simulink model "UAV_sync_known_sim_wrong_version"  (R2018b)
settings: Solver=ode23tb  StartTime=0.0  StopTime=35
values from neighbouring files (symbols this model uses):
  C_rho = 1.225    [SC42120_UAV_Preconditions.m]
  D0 = [M0 0 0 0 0 0 ... (first row only)    [SC42120_UAV_Preconditions.m]
  D1 = [eye(3)*M1 zeros(3,3) ... (first row only)    [UAV_sync_known.m]    (also in UAV_sync_unknown.m; UAV_sync_unknown_gap.m)
  D2 = [eye(3)*M2 zeros(3,3) ... (first row only)    [UAV_sync_known.m]    (also in UAV_sync_unknown.m; UAV_sync_unknown_gap.m)
  Derivative_gain_phi = 50    [SC42120_UAV_Preconditions.m]
  Derivative_gain_psi = 50    [SC42120_UAV_Preconditions.m]
  Derivative_gain_theta = 50    [SC42120_UAV_Preconditions.m]
  Derivative_gain_x = 50    [SC42120_UAV_Preconditions.m]
  Derivative_gain_y = 50    [SC42120_UAV_Preconditions.m]
  Derivative_gain_z = 50    [SC42120_UAV_Preconditions.m]
  G = 9.80665    [SC42120_UAV_Preconditions.m]
  g0 = [0;0;-M0*G;0;0;0]    [SC42120_UAV_Preconditions.m]
  I0 = [0.02 0 -0.01 ... (first row only)    [SC42120_UAV_Preconditions.m]
  I1 = [0.1 0 -0.01 ... (first row only)    [UAV_sync_known.m]    (also in UAV_sync_unknown.m; UAV_sync_unknown_gap.m)
  I2 = 2*[0.1 0 -0.01 ... (first row only)    [UAV_sync_known.m]    (also in UAV_sync_unknown.m; UAV_sync_unknown_gap.m)
  InitWind = [0;0;0]    [SC42120_UAV_Preconditions.m]
  Kp = diag(P)    [SC42120_UAV_Preconditions.m]
  Kv = diag(V)    [SC42120_UAV_Preconditions.m]
  M0 = 10    [SC42120_UAV_Preconditions.m]
  M1 = 20    [UAV_sync_known.m]    (also in UAV_sync_unknown.m; UAV_sync_unknown_gap.m)
  M2 = 30    [UAV_sync_known.m]    (also in UAV_sync_unknown.m; UAV_sync_unknown_gap.m)
  Proportional_phi = 50    [SC42120_UAV_Preconditions.m]
  Proportional_psi = 50    [SC42120_UAV_Preconditions.m]
  Proportional_theta = 50    [SC42120_UAV_Preconditions.m]
  Proportional_x = 50    [SC42120_UAV_Preconditions.m]
  Proportional_y = 50    [SC42120_UAV_Preconditions.m]
  Proportional_z = 50    [SC42120_UAV_Preconditions.m]
undefined symbols (not defined in the file or in its folder): Aero, APlane, Bxl, C, Ctr, deg, DiscIntNeverNeededParam, F, Guid, Init, Light, MIL, Path, rad, s, Trim, Utility
libraries: aerolibconvert2 x37, simulink x15, dspsigops x7, shared6dof x4, aerolibasang x4, sharedutil x4, simulink_extras x3, aerolibadyn x1, aerolibtransform2 x1, aerolibwind2 x1
(part 4 of 6)

== system UAV_sync_known_sim_wrong_version/Node 0/VF Approach/AUTOPILOT/Low-level Controllers/Pitch controller/TRASH ==
  Abs : Abs  Commented=on
  Angle Conversion2 : aerolibconvert2/Angle Conversion  Commented=on  IU=rad  OU=deg
  Angle Conversion3 : aerolibconvert2/Angle Conversion  Commented=on  IU=rad  OU=deg
  Coordination_offset_MATLAB_Fcn : MATLAB Function  Commented=on  TreatAsAtomicUnit=on
  Digital Clock : DigitalClock  Commented=on  SampleTime=0.001
  From : From  Commented=on  GotoTag=roll_ang
  From1 : From  Commented=on  GotoTag=Va  TagVisibility=global
  From2 : From  Commented=on  GotoTag=Va  TagVisibility=global
  From3 : From  Commented=on  GotoTag=pitch_ang
  From5 : From  Commented=on  GotoTag=pitch_ang
  From6 : From  Commented=on  GotoTag=Va  TagVisibility=global
  From7 : From  Commented=on  GotoTag=pitch_ang
  If : If  Commented=on  IfExpression=u1 > 70
  If Action Subsystem : Subsystem  Commented=on  TreatAsAtomicUnit=on
  If Action Subsystem1 : Subsystem  Commented=on  TreatAsAtomicUnit=on
  Merge : Merge  Commented=on
  Parameters mixer1 : Subsystem  Commented=on
  Parameters mixer2 : Subsystem  Commented=on
  Pitch_PID_MATLAB_Fcn : MATLAB Function  Commented=on  TreatAsAtomicUnit=on
  Saturation : Saturate  Commented=on  UpperLimit=80  LowerLimit=-80
  Terminator : Terminator  Commented=on
  wires:
  Parameters mixer2/1(parameters_roll_comp) -> Coordination_offset_MATLAB_Fcn/4(parameters)
  From2/1 -> Coordination_offset_MATLAB_Fcn/3(aspeed)
  From3/1 -> Coordination_offset_MATLAB_Fcn/2(meas_pitch_angle)
  Angle Conversion2/1 -> Coordination_offset_MATLAB_Fcn/1(bank_angle)
  From7/1 -> Abs/1
  Saturation/1 -> If Action Subsystem1/2(bank)
  From5/1 -> If Action Subsystem1/1(pitch)
  From/1 -> Angle Conversion3/1
  If Action Subsystem/1(Out1) -> Merge/1
  If/2 -> If Action Subsystem1/Action
  Angle Conversion3/1 -> Saturation/1
  If/1 -> If Action Subsystem/Action
  Merge/1 -> Terminator/1  "rate offset"
  From6/1 -> If Action Subsystem1/3(Va)
  If Action Subsystem1/1(Out1) -> Merge/2
  Abs/1 -> If/1

== system UAV_sync_known_sim_wrong_version/Node 0/VF Approach/AUTOPILOT/Low-level Controllers/Roll controller/Roll Rate Controller ==
  Desidered rate : Inport
  Roll Rate : Inport  Port=2
  Scaler : Inport  Port=3
  +-45 : Saturate  UpperLimit=45  LowerLimit=-45
  Anti-windup : Subsystem
  Constant4 : Constant  Value=Ctr.Roll.RLL2SRV_I
  Constant8 : Constant  Value=Ctr.Roll.RLL2SRV_D
  Constant9 : Constant  Value=Ctr.TS
  IMAX(deg) : Saturate  UpperLimit=Ctr.Roll.RLL2SRV_IMAX_SCALED  LowerLimit=-Ctr.Roll.RLL2SRV_IMAX_SCALED
  K_FF (real feedforward) : Subsystem
  K_P (feedforward) : Subsystem
  Product2 : Product  Inputs=**
  Product3 : Product  Inputs=****
  Product4 : Product  Inputs=***
  Product5 : Product  Inputs=***
  Product6 : Product  Inputs=***
  Scaler_1 : InportShadow  Port=3
  Scaler_2 : InportShadow  Port=3
  Scaler_3 : InportShadow  Port=3
  Sum2 : Sum  Inputs=|+-
  Sum3 : Sum  Inputs=++++
  Sum5 : Sum  Inputs=++|
  Tau1 : Gain  Gain=Ctr.Roll.RLL2SRV_TCONST
  Unit Delay1 : UnitDelay  SampleTime=Ctr.TS
  Unit Delay2 : UnitDelay  SampleTime=Ctr.TS
  Ail_dem : Outport
  wires:
  Anti-windup/1(y_int) -> Sum5/2
  Product3/1 -> Anti-windup/2(u)  "integrator_delta"
  Unit Delay1/1 -> Sum5/1
  Constant8/1 -> Product5/2
  Product4/1 -> Sum3/2  "PID_P"
  Scaler_3/1 -> Product4/3
  Scaler_2/1 -> Product6/3
  [DesRate] -> Product6/2
  Product2/1 -> [rateErr], Product3/1  "rate_error"
  Roll Rate/1 -> Sum2/2
  Sum2/1 -> Product2/1
  Constant9/1 -> Product3/3
  Scaler/1 -> Product2/2, Product3/4
  IMAX(deg)/1 -> Sum3/1, Unit Delay1/1  "PID_I"
  [rateErr] -> Product5/1
  Product5/1 -> Sum3/3  "PID_D"
  Constant4/1 -> Tau1/1
  Tau1/1 -> Product3/2  "ki_rate"
  Sum3/1 -> Unit Delay2/1, +-45/1
  [DesRate] -> Product4/2
  Scaler_1/1 -> Product5/3
  Product6/1 -> Sum3/4  "PID_FF"
  Unit Delay2/1 -> Anti-windup/1(y)
  Sum5/1 -> IMAX(deg)/1
  +-45/1 -> Ail_dem/1
  Desidered rate/1 -> [DesRate], Sum2/1
  K_P (feedforward)/1(Out1) -> Product4/1
  K_FF (real feedforward)/1(Out1) -> Product6/1

== system UAV_sync_known_sim_wrong_version/Node 0/VF Approach/AUTOPILOT/Low-level Controllers/Roll controller/Roll Rate Controller (simpl. continuous) ==
  Roll Rate Error : Inport
  Roll rate : Inport  Port=2
  Scaler : Inport  Port=3
  Ctr.Roll.RLL2SRV_D : Gain  Gain=Ctr.Roll.RLL2SRV_D
  Integrator : Integrator
  Kp : Gain  Gain=Ctr.Roll.K_P
  Product : Product
  Product1 : Product
  Sum1 : Sum  Inputs=|+-
  Sum2 : Sum  Inputs=+++
  k_I : Gain  Gain=Ctr.Roll.K_I
  AilDemand : Outport
  wires:
  Roll Rate Error/1 -> Sum1/1, Kp/1
  Roll rate/1 -> Sum1/2
  Integrator/1 -> Sum2/3
  Product1/1 -> AilDemand/1
  Product/1 -> k_I/1, Ctr.Roll.RLL2SRV_D/1
  Ctr.Roll.RLL2SRV_D/1 -> Sum2/2
  Sum1/1 -> Product/1
  Scaler/1 -> Product/2, Product1/2
  Kp/1 -> Sum2/1
  k_I/1 -> Integrator/1
  Sum2/1 -> Product1/1

== system UAV_sync_known_sim_wrong_version/Node 0/VF Approach/AUTOPILOT/Low-level Controllers/Side-slip angle controller/Coordination offset ==
  note: Coordinated Turn
  Bank : Inport
  Constant1 : Constant  Value=Ctr.Yaw.YAW2SRV_RLL
  Constant6 : Constant  Value=APlane.airspeed_min
  Constant8 : Constant  Value=C.g
  MinMax : MinMax  Function=max  Inputs=2
  Product1 : Product  Inputs=*/
  Product2 : Product  Inputs=****
  Trigonometric Function : Trigonometry  Operator=tan
  Trigonometric Function1 : Trigonometry  Operator=cos
  yaw_rate_correction : Outport
  wires:
  Constant8/1 -> Product1/1
  [Va] -> MinMax/1
  Constant6/1 -> MinMax/2
  MinMax/1 -> Product1/2
  Product1/1 -> Product2/1
  Trigonometric Function/1 -> Product2/2
  Constant1/1 -> Product2/4
  Bank/1 -> Trigonometric Function1/1, Trigonometric Function/1  "roll angle"
  Trigonometric Function1/1 -> Product2/3
  Product2/1 -> yaw_rate_correction/1

== system UAV_sync_known_sim_wrong_version/Node 0/VF Approach/AUTOPILOT/Low-level Controllers/Side-slip angle controller/High-Pass Filter ==
  note: Highpass filter with cutoff frequency at 0.2 rad/s
  In : Inport
  Gain : Gain  Gain=0.9960080
  Scope : Scope  NumInputPorts=2
  Sum3 : Sum  Inputs=++|
  Sum4 : Sum  Inputs=-+|
  Unit Delay : UnitDelay  SampleTime=Ctr.TS
  Unit Delay1 : UnitDelay  SampleTime=Ctr.TS
  Out : Outport
  wires:
  Unit Delay/1 -> Gain/1
  Sum4/1 -> Sum3/1
  Sum3/1 -> Unit Delay/1, Scope/2, Out/1
  Unit Delay1/1 -> Sum4/1
  Gain/1 -> Sum3/2
  In/1 -> Scope/1, Unit Delay1/1, Sum4/2

== system UAV_sync_known_sim_wrong_version/Node 0/VF Approach/BIXLER DYNAMICS/RUBBISH BIN/Orbit/Chi_d ==
  gamma : Inport
  j : Inport  Port=2
  d : Inport  Port=3
  r : Inport  Port=4
  k : Inport  Port=5
  Vector Field (loiter) : MATLAB Function  TreatAsAtomicUnit=on
  chi_d : Outport
  d_tilde : Outport  Port=2
  wires:
  gamma/1 -> Vector Field (loiter)/1(gamma)
  Vector Field (loiter)/2(d_tilde) -> d_tilde/1
  Vector Field (loiter)/1(chi_d) -> chi_d/1
  k/1 -> Vector Field (loiter)/5(k)
  d/1 -> Vector Field (loiter)/3(d)
  r/1 -> Vector Field (loiter)/4(radius)
  j/1 -> Vector Field (loiter)/2(j)

== system UAV_sync_known_sim_wrong_version/Node 0/VF Approach/BIXLER DYNAMICS/RUBBISH BIN/Orbit/Compute gamma ==
  xy : Inport
  OrbitCenter : Inport  Port=2
  chi : Inport  Port=3
  Demux : Demux  Outputs=2
  L.PolarCoord : MATLAB Function  TreatAsAtomicUnit=on
  Unwrap : dspsigops/Unwrap  tol=pi  running=off
  Zero-Order Hold{2..5} (4 alike) : ZeroOrderHold  SampleTime=-1
  gamma : Outport
  d : Outport  Port=2
  wires:
  Demux/2 -> Zero-Order Hold3/1
  OrbitCenter/1 -> Zero-Order Hold4/1
  L.PolarCoord/2(d) -> d/1
  L.PolarCoord/1(gamma) -> Unwrap/1
  xy/1 -> Demux/1
  Zero-Order Hold2/1 -> L.PolarCoord/1(x)
  Demux/1 -> Zero-Order Hold2/1
  chi/1 -> Zero-Order Hold5/1
  Zero-Order Hold5/1 -> L.PolarCoord/4(chi)
  Zero-Order Hold3/1 -> L.PolarCoord/2(y)
  Zero-Order Hold4/1 -> L.PolarCoord/3(c)
  Unwrap/1 -> gamma/1

== system UAV_sync_known_sim_wrong_version/Node 0/VF Approach/BIXLER DYNAMICS/RUBBISH BIN/Orbit/Extract Vg(xy). ==
  In1 : Inport
  Demux : Demux  Outputs=2
  Math Function : Math  Operator=hypot  SaturateOnIntegerOverflow=on
  Selector3 : Selector  InputPortWidth=3  IndexOptions=Index vector (dialog)  Indices=[1 2]  OutputSizes=1
  Out1 : Outport
  wires:
  In1/1 -> Selector3/1
  Math Function/1 -> Out1/1  "V_g"
  Demux/2 -> Math Function/2
  Selector3/1 -> Demux/1
  Demux/1 -> Math Function/1

== system UAV_sync_known_sim_wrong_version/Node 0/VF Approach/BIXLER DYNAMICS/RUBBISH BIN/Orbit/Loiter Controller ==
  chi : Inport
  chi_d : Inport  Port=2
  d : Inport  Port=3
  Vg_hat : Inport  Port=4
  gamma : Inport  Port=5
  Vg : Inport  Port=6
  param : Inport  Port=7
  Beard Version : MATLAB Function  TreatAsAtomicUnit=on
  Constant : Constant  Value=Guid.Method
  Loiter Controller : MATLAB Function  TreatAsAtomicUnit=on
  Manual Switch1 : ManualSwitch  CurrentSetting=0
  Scope : Scope
  Scope1 : Scope
  Scope10 : Scope  NumInputPorts=2
  Scope4 : Scope
  Switch : Switch  Criteria=u2 > Threshold  Threshold=0.5
  chi:_c : Outport
  wires:
  Loiter Controller/3(beta) -> Scope1/1
  Loiter Controller/5(term3) -> Scope10/2
  Loiter Controller/2(err) -> Scope/1
  Loiter Controller/4(term2) -> Scope10/1, Scope4/1
  chi_d/1 -> Loiter Controller/2(chi_d), [chi_d]
  d/1 -> Beard Version/3(d), Loiter Controller/3(d)
  Vg_hat/1 -> Loiter Controller/4(Vg)
  chi/1 -> Beard Version/1(chi), Loiter Controller/1(chi)
  param/1 -> Beard Version/6(param), Loiter Controller/6(param)
  gamma/1 -> Beard Version/5(gamma), Loiter Controller/5(gamma)
  Constant/1 -> Switch/2
  Loiter Controller/1(y) -> Switch/1
  Beard Version/1(chi_c) -> Switch/3
  Switch/1 -> Manual Switch1/2
  [chi_d] -> Manual Switch1/1
  [chi_d] -> Beard Version/2(chi_d)
  Vg/1 -> Beard Version/4(Vg)
  Manual Switch1/1 -> chi:_c/1

== system UAV_sync_known_sim_wrong_version/Node 0/VF Approach/BIXLER DYNAMICS/RUBBISH BIN/Orbit/Parameters Mixer ==
  Constant1 : Constant  Value=Guid.Est.alpha
  Constant6 : Constant  Value=Guid.Loiter.k
  Constant7 : Constant  Value=Guid.Loiter.kk
  Constant8 : Constant  Value=Guid.Loiter.eps
  Mux : Mux  Inputs=6
  param : Outport
  wires:
  Mux/1 -> param/1
  Constant6/1 -> Mux/1
  Constant7/1 -> Mux/2
  Constant8/1 -> Mux/3
  [R] -> Mux/4
  [j] -> Mux/5
  Constant1/1 -> Mux/6

== system UAV_sync_known_sim_wrong_version/Node 0/VF Approach/BIXLER DYNAMICS/RUBBISH BIN/Orbit/Parameters Mixer1 ==
  Constant : Constant  Value=Guid.Wind.W
  Constant1 : Constant  Value=Guid.Loiter.phiw
  Constant11 : Constant  Value=Guid.Loiter.gamma
  Constant2 : Constant  Value=Guid.Loiter.d_int
  Constant3 : Constant  Value=Guid.Loiter.sigma
  Constant6 : Constant  Value=Guid.Loiter.k
  Constant7 : Constant  Value=Guid.Loiter.kk
  Constant8 : Constant  Value=Guid.Loiter.eps
  Mux : Mux  Inputs=11
  param : Outport
  wires:
  Constant11/1 -> Mux/10
  [R] -> Mux/8
  Mux/1 -> param/1
  [j] -> Mux/9
  Constant/1 -> Mux/1
  Constant8/1 -> Mux/6
  Constant6/1 -> Mux/4
  Constant7/1 -> Mux/5
  [Target_Airspeed] -> Mux/3
  Constant1/1 -> Mux/2
  Constant2/1 -> Mux/7
  Constant3/1 -> Mux/11

== system UAV_sync_known_sim_wrong_version/Node 0/VF Approach/BIXLER DYNAMICS/RUBBISH BIN/Orbit/Vg Estimator ==
  chi : Inport
  d : Inport  Port=2
  gamma : Inport  Port=3
  chi_d : Inport  Port=4
  param : Inport  Port=5
  vg : Inport  Port=6
  Reset : Inport  Port=7
  "Estimator " : MATLAB Function  TreatAsAtomicUnit=on
  Integrator1 : Integrator  ExternalReset=rising  InitialCondition=Guid.Vg0
  Scope16 : Scope  NumInputPorts=4
  Scope17 : Scope  NumInputPorts=3
  Vg_hat : Outport
  wires:
  "Estimator "/1(Vg2_hat_dot) -> Integrator1/1
  "Estimator "/8(chi_tilde) -> Scope17/3
  chi_d/1 -> "Estimator "/5(chi_d)
  "Estimator "/5(term2) -> Scope16/4
  "Estimator "/4(term1) -> Scope16/3
  Integrator1/1 -> Vg_hat/1, [Vg_hat]  "Vg_hat"
  [Vg_hat] -> "Estimator "/3(Vg_hat)
  "Estimator "/7(err_2) -> Scope17/2
  d/1 -> "Estimator "/2(d)
  "Estimator "/6(err_1) -> Scope17/1
  chi/1 -> "Estimator "/1(chi)
  "Estimator "/3(der) -> Scope16/2
  param/1 -> "Estimator "/6(param)
  "Estimator "/2(beta) -> Scope16/1
  gamma/1 -> "Estimator "/4(gamma)
  vg/1 -> "Estimator "/7(Vg)
  Reset/1 -> Integrator1/2

== system UAV_sync_known_sim_wrong_version/Node 0/VF Approach/BIXLER DYNAMICS/RUBBISH BIN/Reference Signals/Pitch Reference Generator ==
  Throttle : Inport
  Angle Conversion1 : aerolibconvert2/Angle Conversion  IU=deg  OU=rad
  "Ctr.Pitch.Trimmed " : Gain  Commented=on  Gain=Ctr.Pitch.Trimmed
  Step1 : Step  Time=Ctr.Gen.stepTimeElev  After=Ctr.Gen.stepElev  SampleTime=0
  Sum : Sum  Inputs=|++
  Pitch Reference : Outport
  wires:
  Step1/1 -> Sum/1
  Angle Conversion1/1 -> Pitch Reference/1  "Pitch Demand (rad)"
  "Ctr.Pitch.Trimmed "/1 -> Sum/2
  Sum/1 -> Angle Conversion1/1
  Throttle/1 -> "Ctr.Pitch.Trimmed "/1

== system UAV_sync_known_sim_wrong_version/Node 0/VF Approach/BIXLER DYNAMICS/RUBBISH BIN/Reference Signals/Roll Reference Generator ==
  Angle Conversion : aerolibconvert2/Angle Conversion  IU=deg  OU=rad
  Scope : Scope
  Step : Step  Commented=on  Time=Ctr.Gen.stepTimeAilFinal  After=-Ctr.Gen.stepAil  SampleTime=0
  Step1 : Step  Time=Ctr.Gen.stepTimeAil  After=Ctr.Gen.stepAil  SampleTime=0
  Step2 : Step  Commented=on  Time=Ctr.Gen.stepTimeAil+Ctr.Gen.stepAilDelay  After=-Ctr.Gen.stepAil  SampleTime=0
  Step3 : Step  Commented=on  Time=Ctr.Gen.stepTimeAilFinal+Ctr.Gen.stepAilDelay  After=Ctr.Gen.stepAil  SampleTime=0
  Sum : Sum  Inputs=++++
  RollDemand : Outport
  wires:
  Step3/1 -> Sum/4
  Step1/1 -> Sum/1
  Step/1 -> Sum/2
  Angle Conversion/1 -> RollDemand/1
  Step2/1 -> Sum/3
  Sum/1 -> Angle Conversion/1, Scope/1

== system UAV_sync_known_sim_wrong_version/Node 0/VF Approach/BIXLER DYNAMICS/RUBBISH BIN/Reference Signals/Yaw Reference Generator ==
  Angle Conversion : aerolibconvert2/Angle Conversion  IU=deg  OU=rad
  Scope : Scope
  Step : Step  Time=Ctr.Gen.stepTimeAilFinal  After=-Ctr.Gen.stepAil  SampleTime=0
  Step1 : Step  Time=Ctr.Gen.stepTimeAil  After=Ctr.Gen.stepAil  SampleTime=0
  Step2 : Step  Time=Ctr.Gen.stepTimeAil+Ctr.Gen.stepAilDelay  After=-Ctr.Gen.stepAil  SampleTime=0
  Step3 : Step  Time=Ctr.Gen.stepTimeAilFinal+Ctr.Gen.stepAilDelay  After=Ctr.Gen.stepAil  SampleTime=0
  Sum : Sum  Inputs=++++
  YawDemand : Outport
  wires:
  Step3/1 -> Sum/4
  Step1/1 -> Sum/1
  Step/1 -> Sum/2
  Angle Conversion/1 -> YawDemand/1
  Step2/1 -> Sum/3
  Sum/1 -> Angle Conversion/1, Scope/1

== system UAV_sync_known_sim_wrong_version/Node 0/VF Approach/BIXLER DYNAMICS/RUBBISH BIN/Reference Signals1/Pitch Reference Generator ==
  Throttle : Inport
  Angle Conversion1 : aerolibconvert2/Angle Conversion  IU=deg  OU=rad
  "Ctr.Pitch.Trimmed " : Gain  Commented=on  Gain=Ctr.Pitch.Trimmed
  Step1 : Step  Time=Ctr.Gen.stepTimeElev  After=Ctr.Gen.stepElev  SampleTime=0
  Sum : Sum  Inputs=|++
  Pitch Reference : Outport
  wires:
  Throttle/1 -> "Ctr.Pitch.Trimmed "/1
  Sum/1 -> Angle Conversion1/1
  "Ctr.Pitch.Trimmed "/1 -> Sum/2
  Angle Conversion1/1 -> Pitch Reference/1  "Pitch Demand (rad)"
  Step1/1 -> Sum/1

== system UAV_sync_known_sim_wrong_version/Node 0/VF Approach/BIXLER DYNAMICS/RUBBISH BIN/Reference Signals1/Roll Reference Generator ==
  Angle Conversion : aerolibconvert2/Angle Conversion  IU=deg  OU=rad
  Scope : Scope
  Step : Step  Commented=on  Time=Ctr.Gen.stepTimeAilFinal  After=-Ctr.Gen.stepAil  SampleTime=0
  Step1 : Step  Time=Ctr.Gen.stepTimeAil  After=Ctr.Gen.stepAil  SampleTime=0
  Step2 : Step  Commented=on  Time=Ctr.Gen.stepTimeAil+Ctr.Gen.stepAilDelay  After=-Ctr.Gen.stepAil  SampleTime=0
  Step3 : Step  Commented=on  Time=Ctr.Gen.stepTimeAilFinal+Ctr.Gen.stepAilDelay  After=Ctr.Gen.stepAil  SampleTime=0
  Sum : Sum  Inputs=++++
  RollDemand : Outport
  wires:
  Sum/1 -> Scope/1, Angle Conversion/1
  Step2/1 -> Sum/3
  Angle Conversion/1 -> RollDemand/1
  Step/1 -> Sum/2
  Step1/1 -> Sum/1
  Step3/1 -> Sum/4

== system UAV_sync_known_sim_wrong_version/Node 0/VF Approach/BIXLER DYNAMICS/RUBBISH BIN/Reference Signals1/Yaw Reference Generator ==
  Angle Conversion : aerolibconvert2/Angle Conversion  IU=deg  OU=rad
  Scope : Scope
  Step : Step  Time=Ctr.Gen.stepTimeAilFinal  After=-Ctr.Gen.stepAil  SampleTime=0
  Step1 : Step  Time=Ctr.Gen.stepTimeAil  After=Ctr.Gen.stepAil  SampleTime=0
  Step2 : Step  Time=Ctr.Gen.stepTimeAil+Ctr.Gen.stepAilDelay  After=-Ctr.Gen.stepAil  SampleTime=0
  Step3 : Step  Time=Ctr.Gen.stepTimeAilFinal+Ctr.Gen.stepAilDelay  After=Ctr.Gen.stepAil  SampleTime=0
  Sum : Sum  Inputs=++++
  YawDemand : Outport
  wires:
  Sum/1 -> Scope/1, Angle Conversion/1
  Step2/1 -> Sum/3
  Angle Conversion/1 -> YawDemand/1
  Step/1 -> Sum/2
  Step1/1 -> Sum/1
  Step3/1 -> Sum/4

== system UAV_sync_known_sim_wrong_version/Node 0/VF Approach/BIXLER DYNAMICS/RUBBISH BIN/Straight Line/Chi_d ==
  ey : Inport
  chi_q : Inport  Port=2
  chi_inf : Inport  Port=3
  k_line : Inport  Port=4
  Vector Field (straight line) : MATLAB Function  TreatAsAtomicUnit=on
  chi_d : Outport
  wires:
  chi_inf/1 -> Vector Field (straight line)/3(chi_inf)
  k_line/1 -> Vector Field (straight line)/4(k_line)
  ey/1 -> Vector Field (straight line)/1(e_y)
  Vector Field (straight line)/1(chi_d) -> chi_d/1
  chi_q/1 -> Vector Field (straight line)/2(chi_q)

== system UAV_sync_known_sim_wrong_version/Node 0/VF Approach/BIXLER DYNAMICS/RUBBISH BIN/Straight Line/Compute crosstrack error ==
  x : Inport
  y : Inport  Port=2
  chi_meas : Inport  Port=3
  SL.Slope : Inport  Port=4
  SL.Line_Origin : Inport  Port=5
  Scope : Scope
  Xtrack error : MATLAB Function  TreatAsAtomicUnit=on
  chi_q : Outport
  e_y : Outport  Port=2  Unit=m
  wires:
  chi_meas/1 -> Xtrack error/3(chi)
  x/1 -> Xtrack error/1(x)
  y/1 -> Xtrack error/2(y)
  Xtrack error/2(epy) -> e_y/1
  SL.Line_Origin/1 -> Xtrack error/5(origin)  "r"
  SL.Slope/1 -> Xtrack error/4(slope)
  Xtrack error/1(chi_q) -> Scope/1, chi_q/1

== system UAV_sync_known_sim_wrong_version/Node 0/VF Approach/BIXLER DYNAMICS/RUBBISH BIN/Straight Line/Extract Vg(xy) ==
  In1 : Inport
  Demux : Demux  Outputs=2
  Math Function : Math  Operator=hypot  SaturateOnIntegerOverflow=on
  Selector3 : Selector  InputPortWidth=3  IndexOptions=Index vector (dialog)  Indices=[1 2]  OutputSizes=1
  Out1 : Outport
  wires:
  Demux/1 -> Math Function/1
  Selector3/1 -> Demux/1
  Demux/2 -> Math Function/2
  Math Function/1 -> Out1/1  "V_g"
  In1/1 -> Selector3/1

== system UAV_sync_known_sim_wrong_version/Node 0/VF Approach/BIXLER DYNAMICS/RUBBISH BIN/Straight Line/Param. Mixer ==
  Constant1 : Constant  Value=Guid.Wind.W
  Constant12 : Constant  Value=Guid.SL.gamma
  Constant2 : Constant  Value=Guid.SL.phiw
  Constant3 : Constant  Value=Guid.SL.eps
  Constant4 : Constant  Value=Guid.SL.epy
  Constant5 : Constant  Value=Guid.SL.sigma
  Constant6 : Constant  Value=Guid.SL.chi_inf
  Constant7 : Constant  Value=Guid.SL.k
  Constant8 : Constant  Value=Guid.SL.kk
  Mux : Mux  Inputs=10
  param : Outport
  wires:
  Mux/1 -> param/1
  Constant4/1 -> Mux/1  "y_int"
  Constant6/1 -> Mux/6  "chi_inf"
  Constant7/1 -> Mux/7  "k"
  Constant1/1 -> Mux/2  "W"
  Constant8/1 -> Mux/8  "kk"
  Constant3/1 -> Mux/4  "epsilon"
  Constant2/1 -> Mux/5  "phiw = constant wind direction"
  Constant12/1 -> Mux/9  "gamma"
  Constant5/1 -> Mux/10  "sigma"
  [Target_Airspeed] -> Mux/3  "Va"

== system UAV_sync_known_sim_wrong_version/Node 0/VF Approach/BIXLER DYNAMICS/RUBBISH BIN/Straight Line/SL.controller ==
  chi : Inport
  chi_d : Inport  Port=2
  e : Inport  Port=3
  Vg_hat : Inport  Port=4
  Vg : Inport  Port=5
  chi_q : Inport  Port=6
  Beard version : MATLAB Function  TreatAsAtomicUnit=on
  Constant : Constant  Value=Guid.Method
  Param. Mixer : Subsystem
  SL.Controller : MATLAB Function  TreatAsAtomicUnit=on
  Switch : Switch  Criteria=u2 > Threshold  Threshold=0.5
  chi_c : Outport
  wires:
  Constant/1 -> Switch/2
  Switch/1 -> chi_c/1
  Param. Mixer/1(param) -> SL.Controller/6(param), Beard version/5(param)
  Vg/1 -> Beard version/4(Vg)
  chi/1 -> Beard version/1(chi), SL.Controller/1(chi)
  chi_d/1 -> Beard version/2(chi_d), SL.Controller/2(chi_d)
  e/1 -> Beard version/3(e), SL.Controller/3(e)
  SL.Controller/1(chi_c) -> Switch/1
  chi_q/1 -> SL.Controller/5(chi_q), Beard version/6(chi_q)
  Beard version/1(chi_c) -> Switch/3
  Vg_hat/1 -> SL.Controller/4(Vg_hat)

== system UAV_sync_known_sim_wrong_version/Node 0/VF Approach/BIXLER DYNAMICS/RUBBISH BIN/Straight Line/Vg Estimator ==
  chi_meas : Inport
  chi_d : Inport  Port=2
  chi_q : Inport  Port=3
  e : Inport  Port=4
  param : Inport  Port=5
  Vg : Inport  Port=6
  Reset : Inport  Port=7
  Integrator : Integrator  ExternalReset=rising  InitialCondition=Guid.Vg0  IgnoreLimit=on
  SL_Estimator : MATLAB Function  TreatAsAtomicUnit=on
  Scope{2,9,11..12} (4 alike) : Scope
  Vg_hat : Outport
  wires:
  param/1 -> SL_Estimator/6(param)
  SL_Estimator/2(e) -> Scope2/1
  SL_Estimator/4(f2) -> Scope11/1
  chi_meas/1 -> SL_Estimator/1(chi)
  SL_Estimator/3(f1) -> Scope9/1
  chi_q/1 -> SL_Estimator/3(chi_q)
  e/1 -> SL_Estimator/4("e ")
  SL_Estimator/1(Vg_hat_dot) -> Integrator/1, Scope12/1
  Integrator/1 -> Vg_hat/1, SL_Estimator/5(Vg_hat)  "Vg2_hat"
  chi_d/1 -> SL_Estimator/2(chi_d)
  Vg/1 -> SL_Estimator/7(Vg)
  Reset/1 -> Integrator/2

== system UAV_sync_known_sim_wrong_version/Node 0/VF Approach/BIXLER DYNAMICS/RUBBISH BIN/TECS/Energy Balance ==
  note: Calculate Specific Energy Balance demand, and the relative errors
  SPE_dem : Inport
  SPE_weighting : Inport  Port=2
  SKE_dem : Inport  Port=3
  SKE_weighting : Inport  Port=4
  SPEdot_dem : Inport  Port=5
  SKEdot_dem : Inport  Port=6
  SPE_est : Inport  Port=7
  SKE_est : Inport  Port=8
  SPEdot_est : Inport  Port=9
  SKEdot_est : Inport  Port=10
  Product{,1..7} (8 alike) : Product
  "SKE_weighting " : InportShadow  Port=4
  SKE_weighting2 : InportShadow  Port=4
  SKE_weighting3 : InportShadow  Port=4
  "SPE_weighting " : InportShadow  Port=2
  "SPE_weighting  " : InportShadow  Port=2
  SPE_weighting2 : InportShadow  Port=2
  Scope : Scope
  Scope1 : Scope
  Scope2 : Scope
  Sum{1..2,4..7} (6 alike) : Sum  Inputs=|+-
  SEB_error : Outport
  SEBdot_dem : Outport  Port=2
  SEBdot_error : Outport  Port=3
  wires:
  Product/1 -> Sum1/1
  SPEdot_est/1 -> Product6/1
  Sum6/1 -> Scope/1, SEBdot_error/1  "SEBdot_error"
  Product6/1 -> Sum7/1
  Product7/1 -> Sum7/2
  SPE_est/1 -> Product4/1
  SPE_weighting2/1 -> Product2/2
  "SKE_weighting "/1 -> Product5/2
  SKE_weighting/1 -> Product1/2
  Product3/1 -> Sum2/2
  Sum1/1 -> Sum4/1  "SEB_dem"
  "SPE_weighting  "/1 -> Product6/2
  Sum5/1 -> Sum4/2
  "SPE_weighting "/1 -> Product4/2
  SKEdot_est/1 -> Product7/1
  SPE_weighting/1 -> Product/2
  Product5/1 -> Sum5/2
  SPEdot_dem/1 -> Product2/1
  SKE_est/1 -> Product5/1
  Sum2/1 -> Scope1/1, SEBdot_dem/1, Sum6/1  "SEBdot_dem"
  SKE_weighting2/1 -> Product3/2
  Product2/1 -> Sum2/1
  Sum4/1 -> Scope2/1, SEB_error/1  "SEB_error"
  Product4/1 -> Sum5/1
  Sum7/1 -> Sum6/2
  SKE_weighting3/1 -> Product7/2
  SKE_dem/1 -> Product1/1
  SPE_dem/1 -> Product/1
  SKEdot_dem/1 -> Product3/1
  Product1/1 -> Sum1/2

== system UAV_sync_known_sim_wrong_version/Node 0/VF Approach/BIXLER DYNAMICS/RUBBISH BIN/TECS/Energy calculations ==
  note: Should be ok
  note: Weighting of the contributes
  PlantData : Inport
  TAS_dem : Inport  Port=2
  HeightDemand : Inport  Port=3
  Bus Creator : BusCreator  Inputs='SPE_weighting','SKE_weighting','SKE_dem','SPE_dem','SPE_est','SKE_est','SKEdot','SPEdot','SKEdot_dem','SPEdot_dem'
  Calculate energies : Subsystem
  Constant3 : Constant  Value=2
  Ctr.TECS.SPDWEIGHT : Constant  Value=Ctr.TECS.SPDWEIGHT
  Saturation1 : Saturate  UpperLimit=2  LowerLimit=0
  Sum3 : Sum  Inputs=|+-
  EnergyBus : Outport
  wires:
  Calculate energies/1(SKE_dem) -> [SKE_dem]
  Calculate energies/8(SKEdot) -> [SKEdot]
  Sum3/1 -> [SPE_weighting]  "SPE_weighting"
  Constant3/1 -> Sum3/1
  TAS_dem/1 -> Calculate energies/1(TAS_dem)
  HeightDemand/1 -> Calculate energies/2(HeightDemand)
  PlantData/1 -> Calculate energies/3(PlantData)
  Saturation1/1 -> [SKE_weighting], Sum3/2  "SKE_weighting"
  Calculate energies/5(SPE_est) -> [SPE_est]
  Calculate energies/7(SPEdot) -> [SPEdot]
  Calculate energies/6(SKE_est) -> [SKE_est]
  Ctr.TECS.SPDWEIGHT/1 -> Saturation1/1
  Calculate energies/2(SKEdot_dem) -> [SKEdot_dem]
  Calculate energies/3(SPE_dem) -> [SPE_dem]
  Calculate energies/4(SPEdot_dem) -> [SPEdot_dem]
  [SPE_weighting] -> Bus Creator/1
  [SKE_weighting] -> Bus Creator/2
  [SKE_dem] -> Bus Creator/3
  [SPE_dem] -> Bus Creator/4
  [SPE_est] -> Bus Creator/5
  [SKE_est] -> Bus Creator/6
  [SKEdot] -> Bus Creator/7
  [SPEdot] -> Bus Creator/8
  [SKEdot_dem] -> Bus Creator/9
  [SPEdot_dem] -> Bus Creator/10
  Bus Creator/1 -> EnergyBus/1

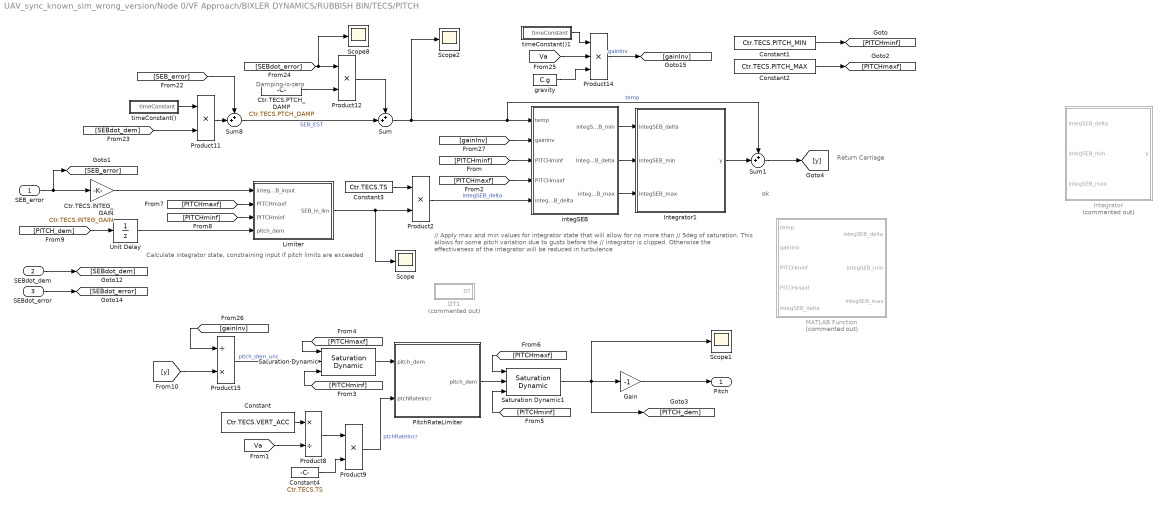
== system UAV_sync_known_sim_wrong_version/Node 0/VF Approach/BIXLER DYNAMICS/RUBBISH BIN/TECS/PITCH ==
  note: ok
  note: Return Carriage
  note: Calculate integrator state, constraining input if pitch limits are exceeded
  note: Damping is zero
  note: // Apply max and min values for integrator state that will allow for no more than
      |     // 5deg of saturation. This allows for some pitch variation due to gusts before the
      |     // integrator is clipped. Otherwise the effectiveness of the integrator will be reduced in turbulence
  SEB_error : Inport
  SEBdot_dem : Inport  Port=2
  SEBdot_error : Inport  Port=3
  Constant : Constant  Value=Ctr.TECS.VERT_ACC
  Constant1 : Constant  Value=Ctr.TECS.PITCH_MIN
  Constant2 : Constant  Value=Ctr.TECS.PITCH_MAX
  Constant3 : Constant  Value=Ctr.TECS.TS
  Constant4 : Constant  Value=Ctr.TECS.TS
  Ctr.TECS.INTEG_GAIN : Gain  Gain=Ctr.TECS.INTEG_GAIN
  Ctr.TECS.PTCH_DAMP : Constant  Value=Ctr.TECS.PTCH_DAMP
  DT1 : Subsystem  Commented=on
  Gain : Gain  Gain=-1
  Integrator : MATLAB Function  Commented=on  TreatAsAtomicUnit=on
  Integrator1 : MATLAB Function  TreatAsAtomicUnit=on
  Limiter : Subsystem
  MATLAB Function : MATLAB Function  Commented=on  TreatAsAtomicUnit=on
  PitchRateLimiter : MATLAB Function  TreatAsAtomicUnit=on
  Product{2,9,11..12} (4 alike) : Product  Inputs=**
  Product14 : Product  Inputs=***
  Product15 : Product  Inputs=/*
  Product8 : Product  Inputs=*/
  Saturation Dynamic : simulink/Discontinuities/Saturation Dynamic  OutMin=[]  OutMax=[]  OutDataTypeStr=Inherit: Same as second input  OutDataType=fixdt(1, 16)  OutScaling=2^-10  DoSatur=off
  Saturation Dynamic1 : simulink/Discontinuities/Saturation Dynamic  OutMin=[]  OutMax=[]  OutDataTypeStr=Inherit: Same as second input  OutDataType=fixdt(1, 16)  OutScaling=2^-10  DoSatur=off
  Scope{,1..2,8} (4 alike) : Scope
  Sum : Sum  Inputs=++|
  Sum1 : Sum  Inputs=++|
  Sum8 : Sum  Inputs=++|
  Unit Delay : UnitDelay  SampleTime=Ctr.TECS.TS
  gravity : Constant  Value=C.g
  integSEB : Subsystem
  timeConstant() : Subsystem
  timeConstant()1 : Subsystem
  Pitch : Outport  Unit=deg
  wires:
  [Va] -> Product8/2
  [SEB_error] -> Sum8/1
  Constant/1 -> Product8/1
  Product9/1 -> PitchRateLimiter/2(ptchRateIncr)  "ptchRateIncr"
  gravity/1 -> Product14/3
  Constant4/1 -> Product9/2
  [SEBdot_dem] -> Product11/2
  Product14/1 -> [gainInv]  "gainInv"
  Product11/1 -> Sum8/2
  Product8/1 -> Product9/1
  Ctr.TECS.PTCH_DAMP/1 -> Product12/2
  [SEBdot_error] -> Scope8/1, Product12/1
  Saturation Dynamic/1 -> PitchRateLimiter/1("pitch_dem ")
  Product15/1 -> Saturation Dynamic/2  "pitch_dem_unc"
  timeConstant()/1(timeConstant) -> Product11/1
  [gainInv] -> Product15/1
  Product12/1 -> Sum/1
  [PITCHminf] -> integSEB/3(PITCHminf)
  [PITCHmaxf] -> integSEB/4(PITCHmaxf)
  PitchRateLimiter/1(pitch_dem) -> Saturation Dynamic1/2
  [Va] -> Product14/2
  timeConstant()1/1(timeConstant) -> Product14/1
  [gainInv] -> integSEB/2(gainInv)
  [PITCHminf] -> Saturation Dynamic/3
  [PITCHmaxf] -> Saturation Dynamic/1
  [PITCHminf] -> Saturation Dynamic1/3
  [PITCHmaxf] -> Saturation Dynamic1/1
  Ctr.TECS.INTEG_GAIN/1 -> Limiter/1(integSEB_input)
  Constant2/1 -> [PITCHmaxf]
  Constant1/1 -> [PITCHminf]
  [PITCHmaxf] -> Limiter/2(PITCHmaxf)
  [PITCHminf] -> Limiter/3(PITCHminf)
  [PITCH_dem] -> Unit Delay/1
  Saturation Dynamic1/1 -> Scope1/1, [PITCH_dem], Gain/1
  Product2/1 -> integSEB/5(integSEB_delta)  "integSEB_delta"
  Constant3/1 -> Product2/1
  Sum8/1 -> Sum/2  "SEB_EST"
  Sum/1 -> Scope2/1, Sum1/1, integSEB/1(temp)  "temp"
  [y] -> Product15/2
  Sum1/1 -> [y]
  Limiter/1(SEB_in_lim) -> Scope/1, Product2/2
  SEB_error/1 -> [SEB_error], Ctr.TECS.INTEG_GAIN/1
  SEBdot_dem/1 -> [SEBdot_dem]
  SEBdot_error/1 -> [SEBdot_error]
  Unit Delay/1 -> Limiter/4(pitch_dem)
  Gain/1 -> Pitch/1
  integSEB/1("integSEB_min ") -> Integrator1/1(integSEB_delta)
  Integrator1/1(y) -> Sum1/2
  integSEB/2("IntegSEB_delta ") -> Integrator1/2(integSEB_min)
  integSEB/3(integSEB_max) -> Integrator1/3(integSEB_max)

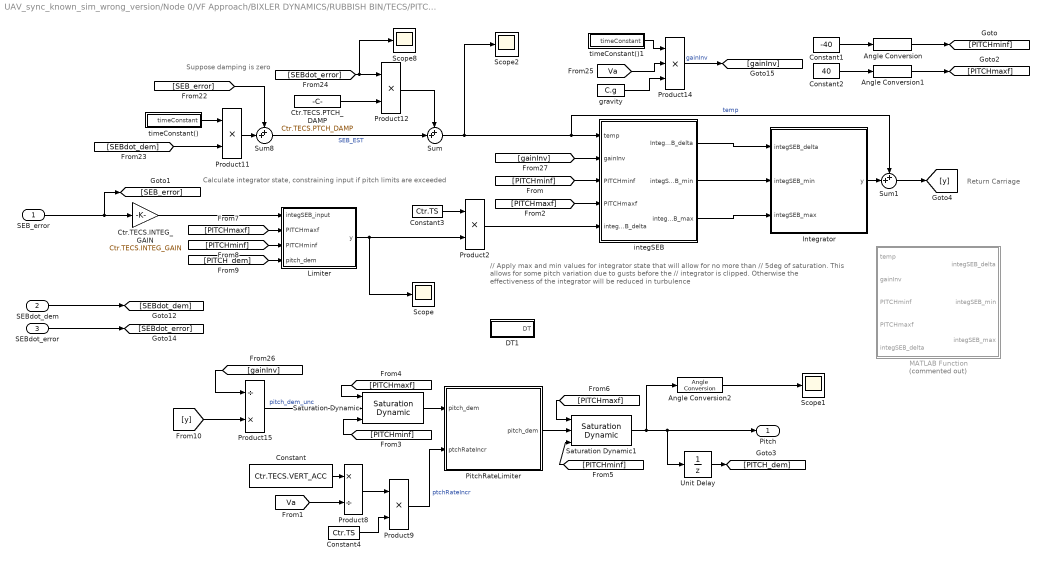
== system UAV_sync_known_sim_wrong_version/Node 0/VF Approach/BIXLER DYNAMICS/RUBBISH BIN/TECS/PITCH1 ==
  note: Return Carriage
  note: Calculate integrator state, constraining input if pitch limits are exceeded
  note: Suppose damping is zero
  note: // Apply max and min values for integrator state that will allow for no more than
      |     // 5deg of saturation. This allows for some pitch variation due to gusts before the
      |     // integrator is clipped. Otherwise the effectiveness of the integrator will be reduced in turbulence
  SEB_error : Inport
  SEBdot_dem : Inport  Port=2
  SEBdot_error : Inport  Port=3
  Angle Conversion : aerolibconvert2/Angle Conversion  IU=deg  OU=rad
  Angle Conversion1 : aerolibconvert2/Angle Conversion  IU=deg  OU=rad
  Angle Conversion2 : aerolibconvert2/Angle Conversion  IU=rad  OU=deg
  Constant : Constant  Value=Ctr.TECS.VERT_ACC
  Constant1 : Constant  Value=-40
  Constant2 : Constant  Value=40
  Constant3 : Constant  Value=Ctr.TS
  Constant4 : Constant  Value=Ctr.TS
  Ctr.TECS.INTEG_GAIN : Gain  Gain=Ctr.TECS.INTEG_GAIN
  Ctr.TECS.PTCH_DAMP : Constant  Value=Ctr.TECS.PTCH_DAMP
  DT1 : Subsystem
  Integrator : MATLAB Function  TreatAsAtomicUnit=on
  Limiter : Subsystem
  MATLAB Function : MATLAB Function  Commented=on  TreatAsAtomicUnit=on
  PitchRateLimiter : MATLAB Function  TreatAsAtomicUnit=on
  Product{2,9,11..12} (4 alike) : Product  Inputs=**
  Product14 : Product  Inputs=***
  Product15 : Product  Inputs=/*
  Product8 : Product  Inputs=*/
  Saturation Dynamic : simulink/Discontinuities/Saturation Dynamic  OutMin=[]  OutMax=[]  OutDataTypeStr=Inherit: Same as second input  OutDataType=fixdt(1, 16)  OutScaling=2^-10  DoSatur=off
  Saturation Dynamic1 : simulink/Discontinuities/Saturation Dynamic  OutMin=[]  OutMax=[]  OutDataTypeStr=Inherit: Same as second input  OutDataType=fixdt(1, 16)  OutScaling=2^-10  DoSatur=off
  Scope{,1..2,8} (4 alike) : Scope
  Sum : Sum  Inputs=++|
  Sum1 : Sum  Inputs=++|
  Sum8 : Sum  Inputs=++|
  Unit Delay : UnitDelay  SampleTime=Ctr.TS
  gravity : Constant  Value=C.g
  integSEB : Subsystem
  timeConstant() : Subsystem
  timeConstant()1 : Subsystem
  Pitch : Outport
  wires:
  [Va] -> Product8/2
  [SEB_error] -> Sum8/1
  Constant/1 -> Product8/1
  Product9/1 -> PitchRateLimiter/2(ptchRateIncr)  "ptchRateIncr"
  gravity/1 -> Product14/3
  Constant4/1 -> Product9/2
  [SEBdot_dem] -> Product11/2
  Product14/1 -> [gainInv]  "gainInv"
  Product11/1 -> Sum8/2
  Product8/1 -> Product9/1
  Ctr.TECS.PTCH_DAMP/1 -> Product12/2
  [SEBdot_error] -> Scope8/1, Product12/1
  Saturation Dynamic/1 -> PitchRateLimiter/1("pitch_dem ")
  Product15/1 -> Saturation Dynamic/2  "pitch_dem_unc"
  timeConstant()/1(timeConstant) -> Product11/1
  [gainInv] -> Product15/1
  Product12/1 -> Sum/1
  [PITCHminf] -> integSEB/3(PITCHminf)
  [PITCHmaxf] -> integSEB/4(PITCHmaxf)
  PitchRateLimiter/1(pitch_dem) -> Saturation Dynamic1/2
  [Va] -> Product14/2
  timeConstant()1/1(timeConstant) -> Product14/1
  [gainInv] -> integSEB/2(gainInv)
  [PITCHminf] -> Saturation Dynamic/3
  [PITCHmaxf] -> Saturation Dynamic/1
  [PITCHminf] -> Saturation Dynamic1/3
  [PITCHmaxf] -> Saturation Dynamic1/1
  Ctr.TECS.INTEG_GAIN/1 -> Limiter/1(integSEB_input)
  Constant1/1 -> Angle Conversion/1
  Constant2/1 -> Angle Conversion1/1
  integSEB/1("IntegSEB_delta ") -> Integrator/1(integSEB_delta)
  Saturation Dynamic1/1 -> Unit Delay/1, Pitch/1, Angle Conversion2/1
  Angle Conversion2/1 -> Scope1/1
  Angle Conversion1/1 -> [PITCHmaxf]
  Angle Conversion/1 -> [PITCHminf]
  [PITCHmaxf] -> Limiter/2(PITCHmaxf)
  [PITCHminf] -> Limiter/3(PITCHminf)
  [PITCH_dem] -> Limiter/4(pitch_dem)
  Unit Delay/1 -> [PITCH_dem]
  Product2/1 -> integSEB/5(integSEB_delta)
  Constant3/1 -> Product2/1
  Sum8/1 -> Sum/2  "SEB_EST"
  Sum/1 -> Scope2/1, Sum1/1, integSEB/1(temp)  "temp"
  integSEB/3(integSEB_max) -> Integrator/3(integSEB_max)
  integSEB/2("integSEB_min ") -> Integrator/2(integSEB_min)
  Integrator/1(y) -> Sum1/2
  [y] -> Product15/2
  Sum1/1 -> [y]
  Limiter/1(y) -> Scope/1, Product2/2
  SEB_error/1 -> [SEB_error], Ctr.TECS.INTEG_GAIN/1
  SEBdot_dem/1 -> [SEBdot_dem]
  SEBdot_error/1 -> [SEBdot_error]

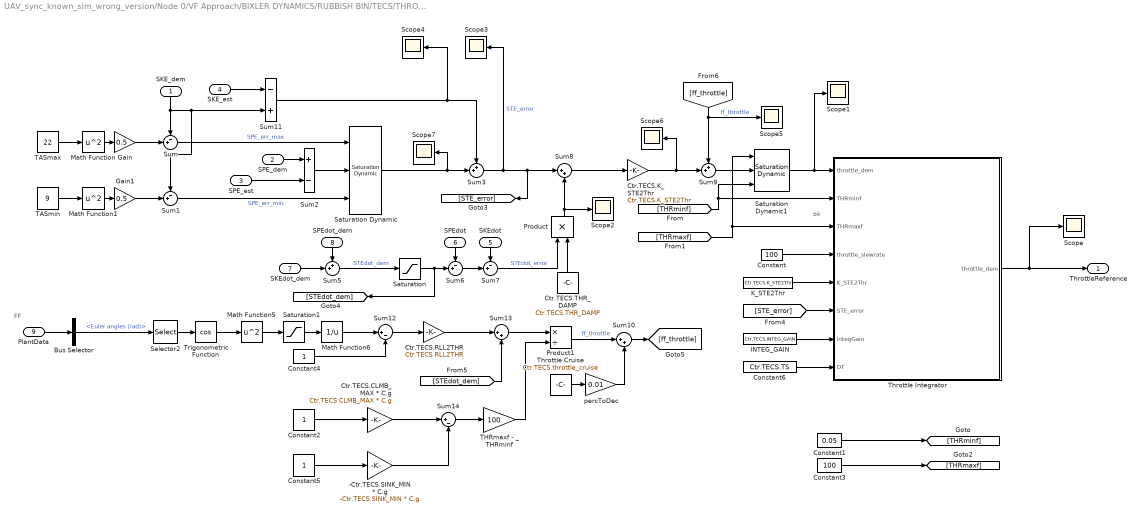
== system UAV_sync_known_sim_wrong_version/Node 0/VF Approach/BIXLER DYNAMICS/RUBBISH BIN/TECS/THROTTLE ==
  note: FF
  note: ok
  SKE_dem : Inport
  SPE_dem : Inport  Port=2
  SPE_est : Inport  Port=3
  SKE_est : Inport  Port=4
  SKEdot : Inport  Port=5
  SPEdot : Inport  Port=6
  SKEdot_dem : Inport  Port=7
  SPEdot_dem : Inport  Port=8
  PlantData : Inport  Port=9
  -Ctr.TECS.SINK_MIN * C.g : Gain  Gain=-Ctr.TECS.SINK_MIN * C.g
  Bus Selector : BusSelector  OutputSignals=Euler angles (rad)
  Constant : Constant  Value=100
  Constant1 : Constant  Value=0.05
  Constant2 : Constant
  Constant3 : Constant  Value=100
  Constant4 : Constant
  Constant5 : Constant
  Constant6 : Constant  Value=Ctr.TECS.TS
  Ctr.TECS.CLMB_MAX * C.g : Gain  Gain=Ctr.TECS.CLMB_MAX * C.g
  Ctr.TECS.K_STE2Thr : Gain  Gain=Ctr.TECS.K_STE2Thr
  Ctr.TECS.RLL2THR : Gain  Gain=Ctr.TECS.RLL2THR
  Ctr.TECS.THR_DAMP : Constant  Value=Ctr.TECS.THR_DAMP
  Gain : Gain  Gain=0.5
  Gain1 : Gain  Gain=0.5
  INTEG_GAIN : Constant  Value=Ctr.TECS.INTEG_GAIN
  K_STE2Thr : Constant  Value=Ctr.TECS.K_STE2Thr
  Math Function : Math  Operator=square  SaturateOnIntegerOverflow=on
  Math Function1 : Math  Operator=square  SaturateOnIntegerOverflow=on
  Math Function5 : Math  Operator=square  SaturateOnIntegerOverflow=on
  Math Function6 : Math  Operator=reciprocal  SaturateOnIntegerOverflow=on
  Product : Product
  Product1 : Product  Inputs=*/
  Saturation : Saturate  UpperLimit=Ctr.TECS.STEdot_max  LowerLimit=Ctr.TECS.STEdot_min
  Saturation Dynamic : simulink/Discontinuities/Saturation Dynamic  OutMin=[]  OutMax=[]  OutDataTypeStr=Inherit: Same as second input  OutDataType=fixdt(1, 16)  OutScaling=2^-10  DoSatur=off
  Saturation Dynamic1 : simulink/Discontinuities/Saturation Dynamic  OutMin=[]  OutMax=[]  OutDataTypeStr=Inherit: Same as second input  OutDataType=fixdt(1, 16)  OutScaling=2^-10  DoSatur=off
  Saturation1 : Saturate  UpperLimit=1  LowerLimit=0.1
  Scope{,1..7} (8 alike) : Scope
  Selector2 : Selector  InputPortWidth=3  IndexOptions=Index vector (dialog)  Indices=1  OutputSizes=1
  Sum{,1,6..7} (4 alike) : Sum  Inputs=-+|
  Sum10 : Sum  Inputs=|++
  Sum11 : Sum  Inputs=-+
  Sum12 : Sum  Inputs=|+-
  Sum13 : Sum  Inputs=|++
  Sum14 : Sum  Inputs=|+-
  Sum2 : Sum  Inputs=+-
  Sum3 : Sum  Inputs=++|
  Sum5 : Sum  Inputs=++|
  Sum8 : Sum  Inputs=|++
  Sum9 : Sum  Inputs=++|
  TASmax : Constant  Value=22
  TASmin : Constant  Value=9
  THRmaxf - _THRminf : Gain  Gain=100
  Throttle Cruise : Constant  Value=Ctr.TECS.throttle_cruise
  Throttle Integrator : MATLAB Function  TreatAsAtomicUnit=on
  Trigonometric Function : Trigonometry  Operator=cos
  percToDec : Gain  Gain=0.01
  ThrottleReference : Outport
  wires:
  Throttle Integrator/1(throttle_dem) -> Scope/1, ThrottleReference/1
  Constant6/1 -> Throttle Integrator/8(DT)
  SKE_dem/1 -> Sum11/2, Sum1/1, Sum/1
  Math Function1/1 -> Gain1/1
  TASmin/1 -> Math Function1/1
  Sum1/1 -> Saturation Dynamic/3  "SPE_err_min"
  Gain1/1 -> Sum1/2
  TASmax/1 -> Math Function/1
  Sum5/1 -> Saturation/1  "STEdot_dem"
  SPEdot/1 -> Sum6/1
  Saturation Dynamic1/1 -> Scope1/1, Throttle Integrator/1("throttle_dem ")
  Product/1 -> Sum8/2, Scope2/1
  Saturation/1 -> [STEdot_dem], Sum6/2
  Ctr.TECS.THR_DAMP/1 -> Product/2
  SPE_est/1 -> Sum2/2
  Sum6/1 -> Sum7/2
  Sum3/1 -> Scope3/1, [STE_error], Sum8/1  "STE_error"
  SPEdot_dem/1 -> Sum5/1
  SKEdot_dem/1 -> Sum5/2
  SKE_est/1 -> Sum11/1
  Sum7/1 -> Product/1  "STEdot_error"
  Sum2/1 -> Saturation Dynamic/2
  SKEdot/1 -> Sum7/1
  Sum9/1 -> Saturation Dynamic1/2
  Sum/1 -> Saturation Dynamic/1  "SPE_err_max"
  Gain/1 -> Sum/2
  Math Function/1 -> Gain/1
  Constant1/1 -> [THRminf]
  Constant3/1 -> [THRmaxf]
  [THRminf] -> Throttle Integrator/2(THRminf), Saturation Dynamic1/3
  [THRmaxf] -> Saturation Dynamic1/1, Throttle Integrator/3(THRmaxf)
  Constant/1 -> Throttle Integrator/4(throttle_slewrate)
  [STE_error] -> Throttle Integrator/6(STE_error)
  INTEG_GAIN/1 -> Throttle Integrator/7(integGain)
  SPE_dem/1 -> Sum2/1
  PlantData/1 -> Bus Selector/1
  Bus Selector/1 -> Selector2/1  "<Euler angles (rad)>"
  Selector2/1 -> Trigonometric Function/1
  Saturation1/1 -> Math Function6/1
  Math Function6/1 -> Sum12/1
  Constant4/1 -> Sum12/2
  Sum12/1 -> Ctr.TECS.RLL2THR/1
  Ctr.TECS.RLL2THR/1 -> Sum13/1
  [STEdot_dem] -> Sum13/2
  Ctr.TECS.K_STE2Thr/1 -> Scope6/1, Sum9/2
  K_STE2Thr/1 -> Throttle Integrator/5(K_STE2Thr)
  [ff_throttle] -> Sum9/1, Scope5/1  "ff_throttle"
  Sum8/1 -> Ctr.TECS.K_STE2Thr/1
  Math Function5/1 -> Saturation1/1
  Sum13/1 -> Product1/1
  Throttle Cruise/1 -> percToDec/1
  Constant2/1 -> Ctr.TECS.CLMB_MAX * C.g/1
  Constant5/1 -> -Ctr.TECS.SINK_MIN * C.g/1
  Ctr.TECS.CLMB_MAX * C.g/1 -> Sum14/1
  -Ctr.TECS.SINK_MIN * C.g/1 -> Sum14/2
  Sum14/1 -> THRmaxf - _THRminf/1
  THRmaxf - _THRminf/1 -> Product1/2
  Product1/1 -> Sum10/1  "ff_throttle"
  Sum10/1 -> [ff_throttle]
  Sum11/1 -> Scope4/1, Sum3/1
  Saturation Dynamic/1 -> Scope7/1, Sum3/2
  percToDec/1 -> Sum10/2
  Trigonometric Function/1 -> Math Function5/1

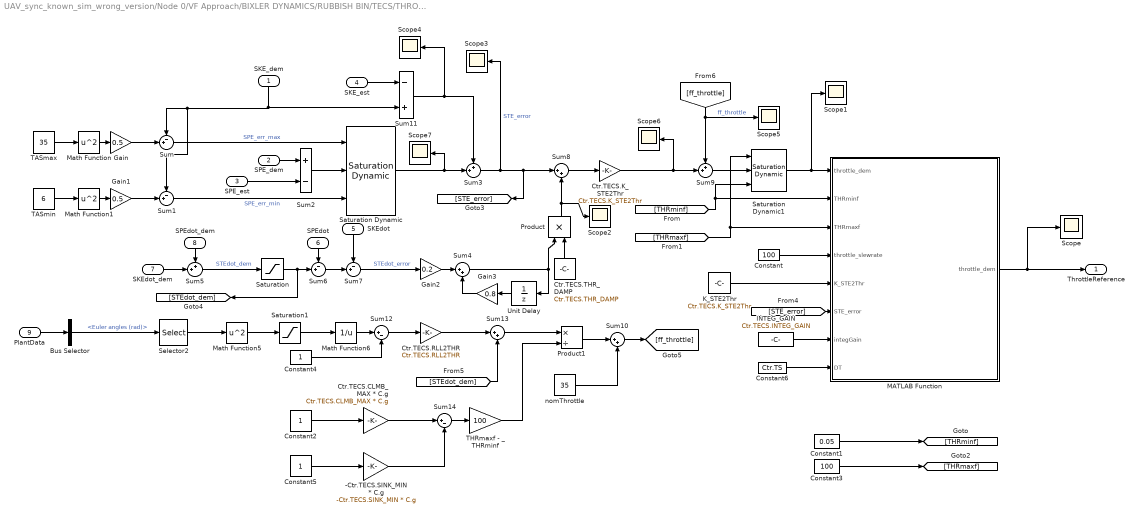
== system UAV_sync_known_sim_wrong_version/Node 0/VF Approach/BIXLER DYNAMICS/RUBBISH BIN/TECS/THROTTLE1 ==
  SKE_dem : Inport
  SPE_dem : Inport  Port=2
  SPE_est : Inport  Port=3
  SKE_est : Inport  Port=4
  SKEdot : Inport  Port=5
  SPEdot : Inport  Port=6
  SKEdot_dem : Inport  Port=7
  SPEdot_dem : Inport  Port=8
  PlantData : Inport  Port=9
  -Ctr.TECS.SINK_MIN * C.g : Gain  Gain=-Ctr.TECS.SINK_MIN * C.g
  Bus Selector : BusSelector  OutputSignals=Euler angles (rad)
  Constant : Constant  Value=100
  Constant1 : Constant  Value=0.05
  Constant2 : Constant
  Constant3 : Constant  Value=100
  Constant4 : Constant
  Constant5 : Constant
  Constant6 : Constant  Value=Ctr.TS
  Ctr.TECS.CLMB_MAX * C.g : Gain  Gain=Ctr.TECS.CLMB_MAX * C.g
  Ctr.TECS.K_STE2Thr : Gain  Gain=Ctr.TECS.K_STE2Thr
  Ctr.TECS.RLL2THR : Gain  Gain=Ctr.TECS.RLL2THR
  Ctr.TECS.THR_DAMP : Constant  Value=Ctr.TECS.THR_DAMP
  Gain : Gain  Gain=0.5
  Gain1 : Gain  Gain=0.5
  Gain2 : Gain  Gain=0.2
  Gain3 : Gain  Gain=0.8
  INTEG_GAIN : Constant  Value=Ctr.TECS.INTEG_GAIN
  K_STE2Thr : Constant  Value=Ctr.TECS.K_STE2Thr
  MATLAB Function : MATLAB Function  TreatAsAtomicUnit=on
  Math Function : Math  Operator=square  SaturateOnIntegerOverflow=on
  Math Function1 : Math  Operator=square  SaturateOnIntegerOverflow=on
  Math Function5 : Math  Operator=square  SaturateOnIntegerOverflow=on
  Math Function6 : Math  Operator=reciprocal  SaturateOnIntegerOverflow=on
  Product : Product
  Product1 : Product  Inputs=*/
  Saturation : Saturate  UpperLimit=Ctr.TECS.STEdot_max  LowerLimit=Ctr.TECS.STEdot_min
  Saturation Dynamic : simulink/Discontinuities/Saturation Dynamic  OutMin=[]  OutMax=[]  OutDataTypeStr=Inherit: Same as second input  OutDataType=fixdt(1, 16)  OutScaling=2^-10  DoSatur=off
  Saturation Dynamic1 : simulink/Discontinuities/Saturation Dynamic  OutMin=[]  OutMax=[]  OutDataTypeStr=Inherit: Same as second input  OutDataType=fixdt(1, 16)  OutScaling=2^-10  DoSatur=off
  Saturation1 : Saturate  UpperLimit=1  LowerLimit=0.1
  Scope{,1..7} (8 alike) : Scope
  Selector2 : Selector  InputPortWidth=3  IndexOptions=Index vector (dialog)  Indices=1  OutputSizes=1
  Sum{,1,6..7} (4 alike) : Sum  Inputs=-+|
  Sum{4,8,10,13} (4 alike) : Sum  Inputs=|++
  Sum11 : Sum  Inputs=-+
  Sum12 : Sum  Inputs=|+-
  Sum14 : Sum  Inputs=|+-
  Sum2 : Sum  Inputs=+-
  Sum3 : Sum  Inputs=++|
  Sum5 : Sum  Inputs=++|
  Sum9 : Sum  Inputs=++|
  TASmax : Constant  Value=35
  TASmin : Constant  Value=6
  THRmaxf - _THRminf : Gain  Gain=100
  Unit Delay : UnitDelay  SampleTime=Ctr.TS
  nomThrottle : Constant  Value=35
  ThrottleReference : Outport
  wires:
  MATLAB Function/1(throttle_dem) -> Scope/1, ThrottleReference/1
  Constant6/1 -> MATLAB Function/8(DT)
  SKE_dem/1 -> Sum/1, Sum1/1, Sum11/2
  Math Function1/1 -> Gain1/1
  TASmin/1 -> Math Function1/1
  Sum1/1 -> Saturation Dynamic/3  "SPE_err_min"
  Gain1/1 -> Sum1/2
  TASmax/1 -> Math Function/1
  Sum5/1 -> Saturation/1  "STEdot_dem"
  SPEdot/1 -> Sum6/1
  Saturation Dynamic1/1 -> Scope1/1, MATLAB Function/1("throttle_dem ")
  Product/1 -> Scope2/1, Sum8/2
  Saturation/1 -> [STEdot_dem], Sum6/2
  Ctr.TECS.THR_DAMP/1 -> Product/2
  SPE_est/1 -> Sum2/2
  Sum6/1 -> Sum7/2
  Sum3/1 -> Scope3/1, [STE_error], Sum8/1  "STE_error"
  SPEdot_dem/1 -> Sum5/1
  SKEdot_dem/1 -> Sum5/2
  SKE_est/1 -> Sum11/1
  Sum7/1 -> Gain2/1  "STEdot_error"
  Sum2/1 -> Saturation Dynamic/2
  SKEdot/1 -> Sum7/1
  Sum9/1 -> Saturation Dynamic1/2
  Sum/1 -> Saturation Dynamic/1  "SPE_err_max"
  Gain/1 -> Sum/2
  Math Function/1 -> Gain/1
  Constant1/1 -> [THRminf]
  Constant3/1 -> [THRmaxf]
  [THRminf] -> MATLAB Function/2(THRminf), Saturation Dynamic1/3
  [THRmaxf] -> Saturation Dynamic1/1, MATLAB Function/3(THRmaxf)
  Constant/1 -> MATLAB Function/4(throttle_slewrate)
  [STE_error] -> MATLAB Function/6(STE_error)
  INTEG_GAIN/1 -> MATLAB Function/7(integGain)
  SPE_dem/1 -> Sum2/1
  PlantData/1 -> Bus Selector/1
  Bus Selector/1 -> Selector2/1  "<Euler angles (rad)>"
  Selector2/1 -> Math Function5/1
  Saturation1/1 -> Math Function6/1
  Math Function6/1 -> Sum12/1
  Constant4/1 -> Sum12/2
  Sum12/1 -> Ctr.TECS.RLL2THR/1
  Ctr.TECS.RLL2THR/1 -> Sum13/1
  [STEdot_dem] -> Sum13/2
  Ctr.TECS.K_STE2Thr/1 -> Scope6/1, Sum9/2
  K_STE2Thr/1 -> MATLAB Function/5(K_STE2Thr)
  [ff_throttle] -> Sum9/1, Scope5/1  "ff_throttle"
  Sum8/1 -> Ctr.TECS.K_STE2Thr/1
  Math Function5/1 -> Saturation1/1
  Sum13/1 -> Product1/1
  nomThrottle/1 -> Sum10/2
  Constant2/1 -> Ctr.TECS.CLMB_MAX * C.g/1
  Constant5/1 -> -Ctr.TECS.SINK_MIN * C.g/1
  Ctr.TECS.CLMB_MAX * C.g/1 -> Sum14/1
  -Ctr.TECS.SINK_MIN * C.g/1 -> Sum14/2
  Sum14/1 -> THRmaxf - _THRminf/1
  THRmaxf - _THRminf/1 -> Product1/2
  Product1/1 -> Sum10/1
  Sum10/1 -> [ff_throttle]
  Sum11/1 -> Scope4/1, Sum3/1
  Gain2/1 -> Sum4/1
  Gain3/1 -> Sum4/2
  Unit Delay/1 -> Gain3/1
  Sum4/1 -> Unit Delay/1, Product/1
  Saturation Dynamic/1 -> Scope7/1, Sum3/2

== system UAV_sync_known_sim_wrong_version/Node 0/VF Approach/BIXLER DYNAMICS/Vehicle Airframe/Aerodynamics/Aerodynamic Coefficients ==
  PlantData : Inport
  Va : Inport  Port=2
  alpha(rad) : Inport  Port=3
  beta(rad) : Inport  Port=4
  Alpha Prelookup : PreLookup  BreakpointsData=Aero.alpha_vector  BeginIndexSearchUsingPreviousIndexResult=on  ExtrapMethod=Linear  RemoveProtectionInput=on
  Angle Conversion : aerolibconvert2/Angle Conversion  IU=rad  OU=deg
  Bus Selector : BusSelector  OutputSignals=Angular rates (body) (rad/s)
  Demux1 : Demux  Outputs=3
  Forces : Subsystem
  Goto Tag Visibility : GotoTagVisibility  GotoTag=pRad
  Goto Tag Visibility1 : GotoTagVisibility  GotoTag=qRad
  Goto Tag Visibility2 : GotoTagVisibility  GotoTag=rRad
  Goto Tag Visibility3 : GotoTagVisibility  GotoTag=BetaRad
  Moments : Subsystem
  Mux : Mux  Inputs=6
  Coeff : Outport
  tag scope: BetaRad=scoped, Va=global, alphaRad=scoped, pRad=scoped, qRad=scoped, rRad=scoped
  wires:
  Alpha Prelookup/2 -> Moments/2(alpha_f), Forces/2(alpha_f)  "f"
  alpha(rad)/1 -> [alphaRad], Angle Conversion/1
  PlantData/1 -> Bus Selector/1
  Forces/1(CD) -> Mux/1
  Forces/2(Cy) -> Mux/2
  Moments/1(Cl) -> Mux/4
  Demux1/3 -> [rRad]  "yaw_rate"
  Angle Conversion/1 -> Alpha Prelookup/1
  Demux1/2 -> [qRad]  "pitch_rate"
  beta(rad)/1 -> [BetaRad]
  Alpha Prelookup/1 -> Moments/1(alpha_k), Forces/1(alpha_k)  "k"
  Demux1/1 -> [pRad]  "roll_rate"
  Forces/3(CL) -> Mux/3
  Moments/3(Cn) -> Mux/6
  Moments/2(Cm) -> Mux/5
  Mux/1 -> Coeff/1
  Bus Selector/1 -> Demux1/1  "<Angular rates (body) (rad/s)>"
  Va/1 -> [Va]

== system UAV_sync_known_sim_wrong_version/Node 0/VF Approach/BIXLER DYNAMICS/Vehicle Airframe/Aerodynamics/ControlIncrements ==
  DerCond : Inport
  Control : Inport  Port=2
  Ailerons : Subsystem
  Alpha : PreLookup  BreakpointsData=Aero.alpha_vector  BeginIndexSearchUsingPreviousIndexResult=on  ExtrapMethod=Linear  RemoveProtectionInput=on
  Angle Conversion : aerolibconvert2/Angle Conversion  IU=rad  OU=deg
  Bus Selector : BusSelector  OutputSignals=alpha
  Bus Selector1 : BusSelector  OutputSignals=delta_ail,delta_elev,delta_rudd
  Elevator : Subsystem
  Rudder : Subsystem
  Cn_ail : Outport
  Cl_ail : Outport  Port=2
  CD_elev : Outport  Port=3
  CL_elev : Outport  Port=4
  Cm_elev : Outport  Port=5
  Cy_rudd : Outport  Port=6
  Cl_rudd : Outport  Port=7
  Cn_rudd : Outport  Port=8
  wires:
  Rudder/3(Cn_rudd) -> Cn_rudd/1
  Rudder/2(Cl_rudd) -> Cl_rudd/1
  Rudder/1(Cy_rudd) -> Cy_rudd/1
  Elevator/3(Cm_elev) -> Cm_elev/1
  Elevator/2(CL_elev) -> CL_elev/1
  Elevator/1(CD_elev) -> CD_elev/1
  Angle Conversion/1 -> Alpha/1
  Ailerons/2(Cl_ail) -> Cl_ail/1
  Ailerons/1(Cn_ail) -> Cn_ail/1
  Bus Selector1/3 -> Rudder/1(deltaRudd)  "<delta_rudd>"
  Bus Selector1/2 -> Elevator/3(DeltaElev)  "<delta_elev>"
  Alpha/2 -> Ailerons/2(alpha_f), Elevator/2(alpha_f)
  Alpha/1 -> Ailerons/1(alpha_k), Elevator/1(alpha_k)
  Bus Selector1/1 -> Ailerons/3(DeltaAil)  "<delta_ail>"
  Bus Selector/1 -> Angle Conversion/1  "<alpha>"
  DerCond/1 -> Bus Selector/1
  Control/1 -> Bus Selector1/1
